simulink library "uav_utilities"  (Simulink 7.1)
values from neighbouring files (symbols this model uses):
  I = find(Ev == Ev(1))    [res_power_junction_m.m]
undefined symbols (not defined in the file or in its folder): euler_0, g, inner_sysd, K_inner, K_outer, Kx_inner, KX_outer, Ky_inner, KY_outer, L, m, omega_0, outer_sysd, pow_gps_pos_sim, pow_gps_vel_sim, pow_imu_pos_sim, pow_imu_rate_sim, pow_sodar_sim, t_comp_inner, t_comp_outer, t_gps, t_imu, t_inner, t_outer, t_sodar, tau, thrust_max, torque_max, Vb_0, XYZ_0
libraries: simulink x33, aero_sim_lib x9, aerolibprivatev1p5 x1
(part 1 of 3)
settings Model: Creator=Administrator  LastModifiedBy=Administrator

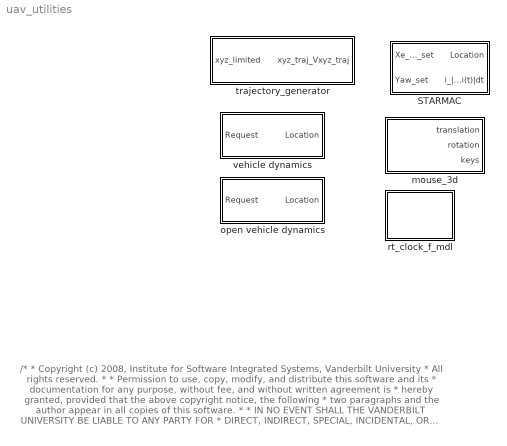
== system uav_utilities ==
  note: /*
      |  * Copyright (c) 2008, Institute for Software Integrated Systems, Vanderbilt University
      |  * All rights reserved.
      |  *
      |  * Permission to use, copy, modify, and distribute this software and its
      |  * documentation for any purpose, without fee, and without written agreement is
      |  * hereby granted, provided that the above copyright notice, the following
      |  * two paragraphs and the author appear in all copies of this software.
      |  *
      |  * IN NO EVENT SHALL THE VANDERBILT UNIVERSITY BE LIABLE TO ANY PARTY FOR
      |  * DIRECT, INDIRECT, SPECIAL, INCIDENTAL, OR CONSEQUENTIAL DAMAGES ARISING OUT
      |  * OF THE USE OF THIS SOFTWARE AND ITS DOCUMENTATION, EVEN IF THE VANDERBILT
      |  * UNIVERSITY HAS BEEN ADVISED OF THE POSSIBILITY OF SUCH DAMAGE.
      |  *
      |  * THE VANDERBILT UNIVERSITY SPECIFICALLY DISCLAIMS ANY WARRANTIES,
      |  * INCLUDING, BUT NOT LIMITED TO, THE IMPLIED WARRANTIES OF MERCHANTABILITY
      |  * AND FITNESS FOR A PARTICULAR PURPOSE.  THE SOFTWARE PROVIDED HEREUNDER IS
      |  * ON AN "AS IS" BASIS, AND THE VANDERBILT UNIVERSITY HAS NO OBLIGATION TO
      |  * PROVIDE MAINTENANCE, SUPPORT, UPDATES, ENHANCEMENTS, OR MODIFICATIONS.
      |  *
      |  * @author Nicholas Kottenstette
      |  */
  STARMAC : Subsystem
  mouse_3d : Subsystem
  open vehicle dynamics : Subsystem  AncestorBlock=uav_utilities/vehicle dynamics
  rt_clock_f_mdl : Subsystem  mask{clock_id=1, T=.01}
      mask prompts: clock_id "Enter clock id (1,2,...) [clock_id]"; T "Enter step time (s) [T]"
      mask init:
      | if clock_id < 1
      |     clock_id = 1;
      | end
      | if T < 0.001
      |     T = .001;
      | end
  trajectory_generator : Subsystem  mask{omega_traj=2*pi/(40*.1), zeta_traj=.9, tau_v_est=.1, T=.01}
      mask prompts: omega_traj "Enter omega trajectory"; zeta_traj "Enter zeta trajectory"; tau_v_est "Enter tau_v_est"; T "Sample time (-1 for inherited):"
      mask init:
      | Hs_x=tf([omega_traj^2],[1 2*zeta_traj*omega_traj omega_traj^2]);
      | Hs_v=tf([1 0],[tau_v_est 1]);
      | Hz_x=ipesh_transform(Hs_x,T);
      | Hz_v=ipesh_transform(Hs_v,T);
  vehicle dynamics : Subsystem

== system uav_utilities/STARMAC ==
  Xe_Ve_set : Inport  PortDimensions=[6]
  Yaw_set : Inport  Port=2  PortDimensions=[1]
  3DM_GX1 : Subsystem  Orientation=left  mask{a_g_s=7000, g_max=5, g_g_s=8500, omega_max=300, Ts=.01}
      mask prompts: a_g_s "AccelGainScale:"; g_max "Max G (1 G = 9.81 m/s^2):"; g_g_s "GyroGainScale:"; omega_max "Mav Angular Velocity (deg/sec):"; Ts "Sample Rate (seconds):"
  Data Type Conversion : DataTypeConversion  OutDataType=sfix(16)  OutScaling=2^0
  Data Type Conversion1 : DataTypeConversion  OutDataType=sfix(16)  OutScaling=2^0
  Demux : Demux  Outputs=[3,3]
  Mux : Mux  Inputs=[3 3 3]
  Rate Transition2 : RateTransition
  SUPERSTAR_II : Subsystem  Orientation=left  mask{Ts=.01}
      mask prompts: Ts "Sample Rate (seconds):"
  Terminator : Terminator
  ZOH : ZeroOrderHold  SampleTime=.01
  ZOH4 : ZeroOrderHold  SampleTime=.01
  Zero-Order Hold : ZeroOrderHold  SampleTime=.02
  dtc : DataTypeConversion  OutDataTypeMode=double  OutDataType=sfix(16)  OutScaling=2^0  OutDataTypeStr=double
  gravity_effects : Constant  Value=zeros(3,1)  OutDataTypeMode=double  OutDataType=sfix(16)  OutScaling=2^0  OutDataTypeStr=double
  gum_stix : Subsystem
  robo_stix : Subsystem  Orientation=left
  starmac_dynamics : Subsystem  AncestorBlock=aero_sim_lib/starmac_dynamics
  Location : Outport
  i_|P_i(t)|dt : Outport  Port=2
  wires:
  ZOH/1 -> Data Type Conversion/1
  robo_stix/5(Ve) -> gum_stix/4(Ve)
  robo_stix/4(Xe) -> gum_stix/3(Xe)
  robo_stix/3(Ab) -> gum_stix/2(Ab)
  Rate Transition2/1 -> dtc/1
  Zero-Order Hold/1 -> Rate Transition2/1
  starmac_dynamics/5(omega) -> 3DM_GX1/3(omega_c)
  dtc/1 -> starmac_dynamics/1(desired_motor_thrust)
  Data Type Conversion/1 -> gum_stix/5(Xe_set)
  gum_stix/2(u_euler) -> robo_stix/4(euler_set)
  gum_stix/1(u_T) -> robo_stix/5(u_T)
  gravity_effects/1 -> starmac_dynamics/2(wind_velocity)
  starmac_dynamics/1(Ve) -> Mux/2, SUPERSTAR_II/2(Ve)  "Ve"
  starmac_dynamics/2(Xe) -> Mux/1, SUPERSTAR_II/1(Xe)  "Xe"
  SUPERSTAR_II/2(Ve_s) -> robo_stix/7(Ve_s)
  SUPERSTAR_II/1(Xe_s) -> robo_stix/6(Xe_s)
  robo_stix/2(euler1) -> gum_stix/1(euler)
  3DM_GX1/3(omega_s) -> robo_stix/3(omega_s)
  3DM_GX1/2(Ab_s) -> robo_stix/2(Ab_s)
  3DM_GX1/1(euler_s) -> robo_stix/1(euler_s)
  starmac_dynamics/7(Ab) -> 3DM_GX1/2(Ab_c)
  starmac_dynamics/3(euler) -> Mux/3, 3DM_GX1/1(euler_c)  "euler"
  robo_stix/1(cont_motor_thrust) -> Zero-Order Hold/1
  Mux/1 -> Location/1
  Xe_Ve_set/1 -> Demux/1
  Demux/1 -> ZOH/1
  Demux/2 -> Terminator/1
  Yaw_set/1 -> ZOH4/1
  ZOH4/1 -> Data Type Conversion1/1
  Data Type Conversion1/1 -> gum_stix/6(Yaw_set)
  starmac_dynamics/8(i_|P_i(t)|dt) -> i_|P_i(t)|dt/1

== system uav_utilities/mouse_3d ==
  Demux : Demux  Outputs=[3,3,-1]
  Gain4 : Gain  Gain=.003  ParameterDataType=sfix(16)  ParameterScaling=2^0  OutDataType=sfix(16)  OutScaling=2^0
  mouse_3d : S-Function  FunctionName=mouse_3d  EnableBusSupport=off
  translation : Outport  OutDataType=sfix(16)  OutScaling=2^0
  rotation : Outport  Port=2  OutDataType=sfix(16)  OutScaling=2^0
  keys : Outport  Port=3  OutDataType=sfix(16)  OutScaling=2^0
  wires:
  Demux/2 -> rotation/1
  Demux/1 -> Gain4/1
  mouse_3d/1 -> Demux/1
  Gain4/1 -> translation/1
  Demux/3 -> keys/1

== system uav_utilities/open vehicle dynamics ==
  note: STARMAC Vehicle Model
  Request : Inport  OutDataType=sfix(16)  OutScaling=2^0
  Angular Rates : ToWorkspace  VariableName=pqr1  SampleTime=-1  SaveFormat=Array
  Body Velocity : ToWorkspace  VariableName=Vb1  SampleTime=-1  SaveFormat=Array
  Clock : Clock
      settings: Decimation=10
  Demux : Demux  Outputs=3
  Demux1 : Demux  Outputs=3
  Demux2 : Demux  Outputs=3
  Demux3 : Demux  Outputs=6
  Euler Angles : ToWorkspace  VariableName=eulerout1  SampleTime=-1  SaveFormat=Array
  Inner Loop : Subsystem
  Mux : Mux  Inputs=9
  Mux1 : Mux  Inputs=3
  Mux2 : Mux  Inputs=3
  Outer Loop Controller : Subsystem
  Position : ToWorkspace  VariableName=xout1  SampleTime=-1  SaveFormat=Array
  Scope : Scope  NumInputPorts=3
      settings: TimeRange=9  YMin=-1~-0.9~-0.65  YMax=1~0.3~0.05  SaveName=ScopeData15  Decimation=10
  Time : ToWorkspace  VariableName=time1  SampleTime=-1  SaveFormat=Array
  Velocity : ToWorkspace  VariableName=vout1  SampleTime=-1  SaveFormat=Array
  Location : Outport  OutDataType=sfix(16)  OutScaling=2^0
  wires:
  Outer Loop Controller/1(Outer Loop Request) -> Inner Loop/1(Outer Loop Request)
  Inner Loop/3(Velocity) -> Outer Loop Controller/3(Velocity), Velocity/1, Demux1/1
  Inner Loop/1(Body vel) -> Body Velocity/1
  Inner Loop/4(Angular Rates) -> Angular Rates/1
  Inner Loop/5(Euler Angles) -> Euler Angles/1, Demux2/1
  Clock/1 -> Time/1
  Inner Loop/6(Inner Loop State) -> Outer Loop Controller/4(Inner Loop  State)
  Demux/1 -> Mux/1
  Demux/2 -> Mux/2
  Demux/3 -> Mux/3
  Demux1/1 -> Mux/4
  Demux1/2 -> Mux/5
  Demux1/3 -> Mux/6
  Demux2/1 -> Mux/7
  Demux2/2 -> Mux/8
  Demux2/3 -> Mux/9
  Demux3/4 -> Mux2/1  "xdot_c"
  Demux3/5 -> Mux2/2  "ydot_c"
  Demux3/6 -> Mux2/3  "zdot_c"
  Demux3/3 -> Mux1/3  "z_c"
  Demux3/1 -> Mux1/1  "x_c"
  Demux3/2 -> Mux1/2  "y_c"
  Mux2/1 -> Scope/1  "speed req"
  Mux1/1 -> Scope/2  "requested location"
  Mux/1 -> Location/1
  Request/1 -> Outer Loop Controller/1(Request), Demux3/1
  Inner Loop/2(Position) -> Position/1, Demux/1, Scope/3, Outer Loop Controller/2(Position)  "curr pos"

== system uav_utilities/rt_clock_f_mdl ==
  force_rate : Scope
      settings: YMin=-7.5  YMax=7.5  SaveName=ScopeData4  MaxDataPoints=100
  rt_clock_f_mdl_in : S-Function  FunctionName=rt_clock_f  Parameters=clock_id,T  EnableBusSupport=off
  wires:
  rt_clock_f_mdl_in/1 -> force_rate/1

== system uav_utilities/trajectory_generator ==
  xyz_limited : Inport  OutDataType=sfix(16)  OutScaling=2^0
  Demux9 : Demux  Outputs=3
  Mux1 : Mux  Inputs=3
  Mux2 : Mux  Inputs=3
  Mux3 : Mux  Inputs=2
  Zero-Order Hold : ZeroOrderHold  SampleTime=T
  Zero-Order Hold1 : ZeroOrderHold  SampleTime=T
  Zero-Order Hold2 : ZeroOrderHold  SampleTime=T
  v_xyz_traj : DiscreteTransferFcn  Numerator=Hz_v.num{1}  Denominator=Hz_v.den{1}  SampleTime=T
  v_xyz_traj1 : DiscreteTransferFcn  Numerator=Hz_v.num{1}  Denominator=Hz_v.den{1}  SampleTime=T
  v_xyz_traj2 : DiscreteTransferFcn  Numerator=Hz_v.num{1}  Denominator=Hz_v.den{1}  SampleTime=T
  xyz_traj : DiscreteTransferFcn  Numerator=Hz_x.num{1}  Denominator=Hz_x.den{1}  SampleTime=T
  xyz_traj1 : DiscreteTransferFcn  Numerator=Hz_x.num{1}  Denominator=Hz_x.den{1}  SampleTime=T
  xyz_traj2 : DiscreteTransferFcn  Numerator=Hz_x.num{1}  Denominator=Hz_x.den{1}  SampleTime=T
  xyz_traj_Vxyz_traj : Outport  OutDataType=sfix(16)  OutScaling=2^0
  wires:
  Mux3/1 -> xyz_traj_Vxyz_traj/1
  Zero-Order Hold2/1 -> Mux3/2
  Zero-Order Hold1/1 -> Mux3/1
  Zero-Order Hold/1 -> Demux9/1
  Mux2/1 -> Zero-Order Hold2/1
  Mux1/1 -> Zero-Order Hold1/1
  xyz_limited/1 -> Zero-Order Hold/1
  v_xyz_traj2/1 -> Mux2/3
  v_xyz_traj/1 -> Mux2/1
  v_xyz_traj1/1 -> Mux2/2
  xyz_traj2/1 -> Mux1/3, v_xyz_traj2/1
  xyz_traj1/1 -> Mux1/2, v_xyz_traj1/1
  xyz_traj/1 -> Mux1/1, v_xyz_traj/1
  Demux9/3 -> xyz_traj2/1
  Demux9/2 -> xyz_traj1/1
  Demux9/1 -> xyz_traj/1

== system uav_utilities/vehicle dynamics ==
  note: STARMAC Vehicle Model
  Request : Inport
  Angular Rates : ToWorkspace  VariableName=pqr1  SampleTime=-1  SaveFormat=Array
  Body Velocity : ToWorkspace  VariableName=Vb1  SampleTime=-1  SaveFormat=Array
  Clock : Clock
      settings: Decimation=10
  Demux : Demux  Outputs=3
  Demux1 : Demux  Outputs=3
  Demux2 : Demux  Outputs=3
  Demux3 : Demux  Outputs=6
  Euler Angles : ToWorkspace  VariableName=eulerout1  SampleTime=-1  SaveFormat=Array
  Inner Loop : Subsystem
  Mux : Mux  Inputs=9
  Mux1 : Mux  Inputs=3
  Mux2 : Mux  Inputs=3
  Outer Loop Controller : Subsystem
  Position : ToWorkspace  VariableName=xout1  SampleTime=-1  SaveFormat=Array
  Scope : Scope  NumInputPorts=3
      settings: TimeRange=9  YMin=-1~-0.9~-0.65  YMax=1~0.3~0.05  SaveName=ScopeData15  Decimation=10
  Time : ToWorkspace  VariableName=time1  SampleTime=-1  SaveFormat=Array
  Velocity : ToWorkspace  VariableName=vout1  SampleTime=-1  SaveFormat=Array
  Location : Outport
  wires:
  Inner Loop/2(Position) -> Outer Loop Controller/2(Position), Scope/3, Demux/1, Position/1  "curr pos"
  Request/1 -> Demux3/1, Outer Loop Controller/1(Request)
  Mux/1 -> Location/1
  Mux1/1 -> Scope/2  "requested location"
  Mux2/1 -> Scope/1  "speed req"
  Demux3/2 -> Mux1/2  "y_c"
  Demux3/1 -> Mux1/1  "x_c"
  Demux3/3 -> Mux1/3  "z_c"
  Demux3/6 -> Mux2/3  "zdot_c"
  Demux3/5 -> Mux2/2  "ydot_c"
  Demux3/4 -> Mux2/1  "xdot_c"
  Demux2/3 -> Mux/9
  Demux2/2 -> Mux/8
  Demux2/1 -> Mux/7
  Demux1/3 -> Mux/6
  Demux1/2 -> Mux/5
  Demux1/1 -> Mux/4
  Demux/3 -> Mux/3
  Demux/2 -> Mux/2
  Demux/1 -> Mux/1
  Inner Loop/6(Inner Loop State) -> Outer Loop Controller/4(Inner Loop  State)
  Clock/1 -> Time/1
  Inner Loop/5(Euler Angles) -> Demux2/1, Euler Angles/1
  Inner Loop/4(Angular Rates) -> Angular Rates/1
  Inner Loop/1(Body vel) -> Body Velocity/1
  Inner Loop/3(Velocity) -> Demux1/1, Velocity/1, Outer Loop Controller/3(Velocity)
  Outer Loop Controller/1(Outer Loop Request) -> Inner Loop/1(Outer Loop Request)

== system uav_utilities/STARMAC/3DM_GX1 ==
  euler_c : Inport  Orientation=left
  Ab_c : Inport  Orientation=left  Port=2
  omega_c : Inport  Orientation=left  Port=3
  Demux : Demux  Orientation=left  Outputs=[3 3 3]
  Mux : Mux  Orientation=left  Inputs=[3 3 3]
  Quantizer : Quantizer  Orientation=left  QuantizationInterval=pi/(2^15)*ones(3,1)
  Quantizer1 : Quantizer  Orientation=left  QuantizationInterval=g_max*9.81/(2^15)*ones(3,1)
  Quantizer2 : Quantizer  Orientation=left  QuantizationInterval=(pi*omega_max/180)/(2^15)*ones(3,1)
  Saturation : Saturate  Orientation=left  UpperLimit=((2^15)-1)*ones(3,1)  LowerLimit=-(2^15)*ones(3,1)  OutDataType=sfix(16)  OutScaling=2^0
  Saturation1 : Saturate  Orientation=left  UpperLimit=((2^15)-1)*ones(3,1)  LowerLimit=-(2^15)*ones(3,1)  OutDataType=sfix(16)  OutScaling=2^0
  Zero-Order Hold : ZeroOrderHold  Orientation=left  SampleTime=Ts
  counts_per_accel : Gain  Orientation=left  Gain=1e3*(2^15)/(9.81*a_g_s)  ParameterDataType=sfix(16)  ParameterScaling=2^0  OutDataType=sfix(16)  OutScaling=2^0
  counts_per_radian : Gain  Orientation=left  Gain=(2^15)/pi  ParameterDataType=sfix(16)  ParameterScaling=2^0  OutDataType=sfix(16)  OutScaling=2^0
  counts_per_radian_p_sec : Gain  Orientation=left  Gain=1e3*(2^15)/g_g_s  ParameterDataType=sfix(16)  ParameterScaling=2^0  OutDataType=sfix(16)  OutScaling=2^0
  dtc1 : DataTypeConversion  Orientation=left  OutDataTypeMode=single  OutDataType=sfix(16)  OutScaling=2^0  OutDataTypeStr=single
  dtc2 : DataTypeConversion  Orientation=left  OutDataTypeMode=single  OutDataType=sfix(16)  OutScaling=2^0  OutDataTypeStr=single
  dtc3 : DataTypeConversion  Orientation=left  OutDataTypeMode=single  OutDataType=sfix(16)  OutScaling=2^0  OutDataTypeStr=single
  euler_s : Outport  Orientation=left
  Ab_s : Outport  Orientation=left  Port=2
  omega_s : Outport  Orientation=left  Port=3
  wires:
  counts_per_radian/1 -> dtc1/1
  dtc3/1 -> omega_s/1
  dtc2/1 -> Ab_s/1
  dtc1/1 -> euler_s/1
  Saturation1/1 -> dtc3/1
  Saturation/1 -> dtc2/1
  Quantizer2/1 -> counts_per_radian_p_sec/1
  counts_per_radian_p_sec/1 -> Saturation1/1
  Demux/3 -> Quantizer2/1
  counts_per_accel/1 -> Saturation/1
  Quantizer1/1 -> counts_per_accel/1
  Quantizer/1 -> counts_per_radian/1
  Demux/2 -> Quantizer1/1
  Demux/1 -> Quantizer/1
  Zero-Order Hold/1 -> Demux/1
  omega_c/1 -> Mux/3
  Ab_c/1 -> Mux/2
  euler_c/1 -> Mux/1
  Mux/1 -> Zero-Order Hold/1

== system uav_utilities/STARMAC/SUPERSTAR_II ==
  Xe : Inport  Orientation=left
  Ve : Inport  Orientation=left  Port=2
  Demux : Demux  Orientation=left  Outputs=[3 3]
  Mux : Mux  Orientation=left  Inputs=[3 3]
  Rate Transition : RateTransition  Orientation=left
  ZOH : ZeroOrderHold  Orientation=left  SampleTime=Ts
  dtc1 : DataTypeConversion  Orientation=left  OutDataTypeMode=single  OutDataType=sfix(16)  OutScaling=2^0  OutDataTypeStr=single
  dtc2 : DataTypeConversion  Orientation=left  OutDataTypeMode=single  OutDataType=sfix(16)  OutScaling=2^0  OutDataTypeStr=single
  Xe_s : Outport  Orientation=left
  Ve_s : Outport  Orientation=left  Port=2
  wires:
  Rate Transition/1 -> Demux/1
  dtc2/1 -> Ve_s/1
  dtc1/1 -> Xe_s/1
  Demux/2 -> dtc2/1
  Demux/1 -> dtc1/1
  Mux/1 -> ZOH/1
  Xe/1 -> Mux/1
  Ve/1 -> Mux/2
  ZOH/1 -> Rate Transition/1

== system uav_utilities/STARMAC/gum_stix ==
  euler : Inport  PortDimensions=[3]  DataType=single  OutDataTypeStr=single
  Ab : Inport  Port=2  PortDimensions=[3]  DataType=single  OutDataTypeStr=single
  Xe : Inport  Port=3  PortDimensions=[3]  DataType=single  OutDataTypeStr=single
  Ve : Inport  Port=4  PortDimensions=[3]  DataType=single  OutDataTypeStr=single
  Xe_set : Inport  Port=5  PortDimensions=[3]  DataType=single  OutDataTypeStr=single
  Yaw_set : Inport  Port=6  PortDimensions=[1]  DataType=single  OutDataTypeStr=single
  Demux : Demux  Outputs=3
  body_to_inertial : Subsystem
  inertial_pos_controller : Subsystem
  rate_limiter : Subsystem  mask{wn=2*pi, zeta=0.9, Vmax=2, T=0.01}
      mask prompts: wn "omega_n"; Vmax "Max velocity"; T "Sample time"
      mask init:
      | Hs=tf([wn^2],[1,2*zeta*wn,wn^2]);
      | Hz=ipesh_transform(Hs,T);
  sc1 : Scope
      settings: YMin=-7.5  YMax=22.5  SaveName=ScopeData8  Decimation=10
  sc2 : Scope
      settings: YMin=-2  YMax=2  SaveName=ScopeData9  Decimation=10
  sensor_fusion : Subsystem
  u_T : Outport  PortDimensions=[1]  DataType=single  OutDataTypeStr=single
  u_euler : Outport  Port=2  PortDimensions=[3]  DataType=single  OutDataTypeStr=single
  wires:
  Yaw_set/1 -> inertial_pos_controller/5(Yaw_set)
  Demux/3 -> inertial_pos_controller/4(Yaw_actual)
  rate_limiter/1(Xr_set) -> sc2/1, inertial_pos_controller/1(Xe_set)
  Ve/1 -> sensor_fusion/4(Ve_s)
  Xe/1 -> sensor_fusion/3(Xe_s)
  body_to_inertial/2(Ve) -> sensor_fusion/2(Ve_f)
  body_to_inertial/1(Xe) -> sensor_fusion/1(Xe_f)
  sensor_fusion/2(Ve) -> inertial_pos_controller/3(Ve)
  sensor_fusion/1(Xe) -> inertial_pos_controller/2(Xe)
  Ab/1 -> body_to_inertial/2(Ab)
  euler/1 -> Demux/1, body_to_inertial/1(euler)
  inertial_pos_controller/2(u_euler) -> u_euler/1
  inertial_pos_controller/1(u_T) -> u_T/1
  Xe_set/1 -> sc1/1, rate_limiter/1(Xe_set)

== system uav_utilities/STARMAC/robo_stix ==
  euler_s : Inport  PortDimensions=[3]  DataType=single  OutDataTypeStr=single
  Ab_s : Inport  Port=2  PortDimensions=[3]  DataType=single  OutDataTypeStr=single
  omega_s : Inport  Port=3  PortDimensions=[3]  DataType=single  OutDataTypeStr=single
  euler_set : Inport  Port=4  PortDimensions=[3]  DataType=single  OutDataTypeStr=single
  u_T : Inport  Port=5  PortDimensions=[1]  DataType=single  OutDataTypeStr=single
  Xe_s : Inport  Port=6  PortDimensions=[3]  DataType=single  OutDataTypeStr=single
  Ve_s : Inport  Port=7  PortDimensions=[3]  DataType=single  OutDataTypeStr=single
  euler_controller : Subsystem  mask{K=1, K_e=7.5/.65, K_o=.5}
      mask prompts: K "Loop Gain [K]:"; K_e "Euler Gain [K_e]:"; K_o "Omega Gain [K_o]:"
  lead_motor : Subsystem  mask{tau_motor=.10, t_s=.01}
      mask init:
      | Hs=tf([tau_motor 1],[t_s/pi 1]);
      | Hz=ipesh_transform(Hs,t_s);
      | %a=1/tau_motor;
      | %b=pi/t_s;
      | %T=t_s;
      | %num1=b*(1-exp(-b*T))+a*(b*T-1+exp(-b*T));
      | %num2=-b*(1-exp(-b*T))+a*(1-exp(-b*T)-b*T*exp(-b*T));
      | %den1=a*b;
      | %den2=-a*b*exp(-b*T);
      | %num=[num1 num2];
      | %den=[den1 den2];
      | %Hz=tf(num,den,T);
      | %[y,t]=step(Hz);
      | %k_ss=(1/y(length(y)));
      | %num=k_ss*num;
      | %lead_a_1=single(-den(2)/den(1))
      | %lead_b_1=single(num(2)/den(1))
      | %lead_b_2=single(num(1)/den(1))
      | %Hz=k_ss*Hz
      | %bode(Hz);
  sensor_convert : Subsystem  mask{a_g_s=7000, g_g_s=8500}
      mask prompts: a_g_s "AccelGainScale[a_g_s]:"; g_g_s "GyroGainScale[g_g_s]:"
  thrust_limit : Saturate  UpperLimit=10*ones(4,1)  LowerLimit=0*ones(4,1)  OutDataTypeMode=single  OutDataType=sfix(16)  OutScaling=2^0  OutDataTypeStr=single
  u_T_u_torque_motor_thrust : Subsystem  mask{dx=.3048, K_torque=.47}
      mask prompts: dx "X distance of motor from CG [dx](meters):"; K_torque "Ktorque [K_torque]:"
      mask init:
      | M=[0 -dx 0 dx;
      |    dx 0 -dx 0;
      |    -K_torque K_torque -K_torque K_torque;
      |    1 1 1 1];
      | Mi=single(inv(M));
  cont_motor_thrust : Outport
  euler1 : Outport  Port=2
  Ab : Outport  Port=3
  Xe : Outport  Port=4
  Ve : Outport  Port=5
  wires:
  lead_motor/1(thrust_out) -> thrust_limit/1
  u_T_u_torque_motor_thrust/1(cont_motor_thrust) -> lead_motor/1(thrust_in)
  Xe_s/1 -> Xe/1
  thrust_limit/1 -> cont_motor_thrust/1
  Ve_s/1 -> Ve/1
  sensor_convert/2(Ab) -> Ab/1
  euler_controller/1(u_torque) -> u_T_u_torque_motor_thrust/1(u_torque)
  u_T/1 -> u_T_u_torque_motor_thrust/2(u_T)
  sensor_convert/3(omega) -> euler_controller/3(omega)
  euler_set/1 -> euler_controller/1(euler_set)
  sensor_convert/1(euler) -> euler1/1, euler_controller/2(euler)
  omega_s/1 -> sensor_convert/3(omega_s)
  Ab_s/1 -> sensor_convert/2(Ab_s)
  euler_s/1 -> sensor_convert/1(euler_s)

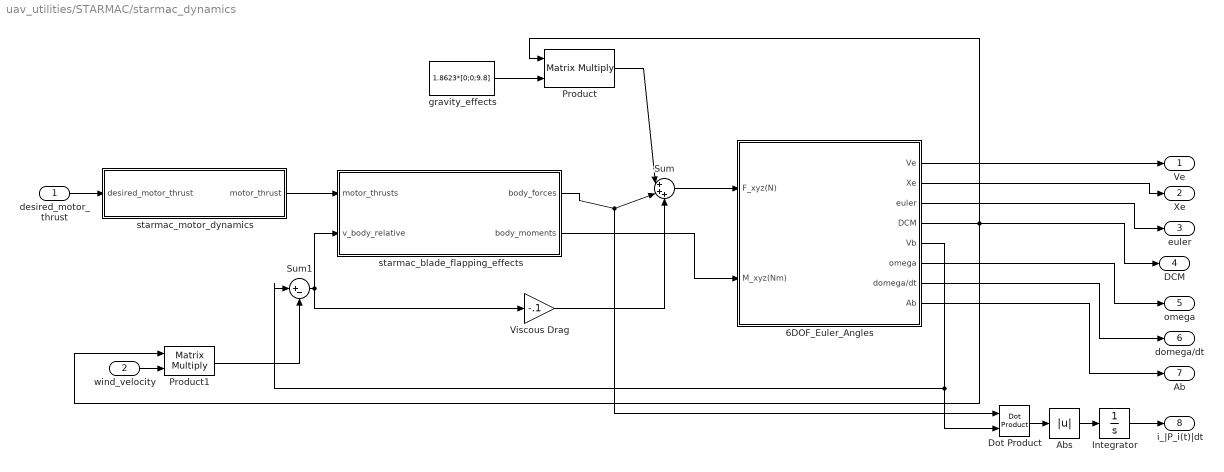
== system uav_utilities/STARMAC/starmac_dynamics ==
  desired_motor_thrust : Inport  OutDataType=sfix(16)  OutScaling=2^0
  wind_velocity : Inport  Port=2  OutDataType=sfix(16)  OutScaling=2^0
  6DOF_Euler_Angles : Subsystem  AncestorBlock=aero_sim_lib/6DOF (Euler Angles)_CMU  mask{XYZe_0=[0.1;0.2;0], Vb_0=[0;0;0], euler_0=[0;0;0], omega_0=[0;0;0], M=1.8623, I=diag([0.02759 0.02771 0.04806])}
      mask prompts: XYZe_0 "Initial position in inertial axes [Xe,Ye,Ze]:"; Vb_0 "Initial velocity in body axes [U,v,w]:"; euler_0 "Initial Euler orientation [roll, pitch, yaw]=[phi,theta,psi]:"; omega_0 "Initial body rotation rates [p,q,r]=omega:"; M "Initial mass:"; I "Inertial:"
  Abs : Abs  OutDataType=sfix(16)  OutScaling=2^0
  Dot Product : simulink/Math Operations/Dot Product  InputSameDT=on  OutDataType=sfix(16)  OutScaling=2^-10  DoSatur=off
  Integrator : Integrator
  Product : Product  Multiplication=Matrix(*)  OutDataType=sfix(16)  OutScaling=2^0  RndMeth=Zero
  Product1 : Product  Multiplication=Matrix(*)  OutDataType=sfix(16)  OutScaling=2^0  RndMeth=Zero
  Sum : Sum  Inputs=|+++  OutDataType=sfix(16)  OutScaling=2^0
  Sum1 : Sum  Inputs=|+-  OutDataType=sfix(16)  OutScaling=2^0
  Viscous Drag : Gain  Gain=-.1  ParameterDataType=sfix(16)  ParameterScaling=2^0  OutDataType=sfix(16)  OutScaling=2^0
  gravity_effects : Constant  Value=1.8623*[0;0;9.8]  OutDataType=sfix(16)  OutScaling=2^0
  starmac_blade_flapping_effects : Subsystem  AncestorBlock=aero_sim_lib/starmac_blade_flapping_effects
  starmac_motor_dynamics : Subsystem  AncestorBlock=aero_sim_lib/starmac_motor_dynamics  mask{tau_motor=.1, T_nom=1.8263*9.8/4, thrust_max=9.8, thrust_min=0, motor_lag_enable=on, motor_variance=.01*(.05*9.8/4)^2, Ts=1/76}
      mask prompts: tau_motor "tau_motor (seconds):"; T_nom "nominal thrust (N):"; thrust_max "maximum thrust (N):"; thrust_min "minimum thrust (N):"; motor_lag_enable "Motor Lag Enabled:"; motor_variance "Motor Variance [motor_variance]:"; Ts "Motor Update Rate (seconds):"
  Ve : Outport  OutDataType=sfix(16)  OutScaling=2^0
  Xe : Outport  Port=2  OutDataType=sfix(16)  OutScaling=2^0
  euler : Outport  Port=3  OutDataType=sfix(16)  OutScaling=2^0
  DCM : Outport  Port=4  OutDataType=sfix(16)  OutScaling=2^0
  omega : Outport  Port=5  OutDataType=sfix(16)  OutScaling=2^0
  domega/dt : Outport  Port=6  OutDataType=sfix(16)  OutScaling=2^0
  Ab : Outport  Port=7  OutDataType=sfix(16)  OutScaling=2^0
  i_|P_i(t)|dt : Outport  Port=8  OutDataType=sfix(16)  OutScaling=2^0
  wires:
  Abs/1 -> Integrator/1
  Dot Product/1 -> Abs/1
  Integrator/1 -> i_|P_i(t)|dt/1
  6DOF_Euler_Angles/8(Ab) -> Ab/1
  6DOF_Euler_Angles/7(domega/dt) -> domega/dt/1
  6DOF_Euler_Angles/6(omega) -> omega/1
  6DOF_Euler_Angles/3(euler) -> euler/1
  6DOF_Euler_Angles/2(Xe) -> Xe/1
  6DOF_Euler_Angles/1(Ve) -> Ve/1
  starmac_motor_dynamics/1(motor_thrust) -> starmac_blade_flapping_effects/1(motor_thrusts)
  Product/1 -> Sum/1
  Sum/1 -> 6DOF_Euler_Angles/1(F_xyz(N))
  6DOF_Euler_Angles/4(DCM) -> DCM/1, Product/1, Product1/1
  gravity_effects/1 -> Product/2
  Sum1/1 -> starmac_blade_flapping_effects/2(v_body_relative), Viscous Drag/1
  Product1/1 -> Sum1/2
  6DOF_Euler_Angles/5(Vb) -> Dot Product/2, Sum1/1
  Viscous Drag/1 -> Sum/3
  starmac_blade_flapping_effects/2(body_moments) -> 6DOF_Euler_Angles/2(M_xyz(Nm))
  starmac_blade_flapping_effects/1(body_forces) -> Dot Product/1, Sum/2
  desired_motor_thrust/1 -> starmac_motor_dynamics/1(desired_motor_thrust)
  wind_velocity/1 -> Product1/2

== system uav_utilities/open vehicle dynamics/Inner Loop ==
  note: Inner Loop Model
  note: \phi,\theta,\psi,p,q,r
  note: \phi,\theta,\psi
  Outer Loop Request : Inport  OutDataType=sfix(16)  OutScaling=2^0
  Attitude Request : ToWorkspace  VariableName=eulreq1  SampleTime=-1  SaveFormat=Array
  Demux1 : Demux  Orientation=left  Outputs=3
  Inner Loop Controller : Subsystem
  Mux1 : Mux  Orientation=left  Inputs=2
  Non-Linear Dynamics : Subsystem
  Saturation : Subsystem
  attitude : Scope
      settings: YMin=-4  YMax=10  SaveName=ScopeData4
  pqr : Scope
      settings: YMin=-4  YMax=10  SaveName=ScopeData3
  velocity : Scope
      settings: YMin=-4  YMax=10  SaveName=ScopeData2
  x : Terminator
  xyz : Scope
      settings: YMin=-0.1  YMax=1.2
  y : Terminator
  Body vel : Outport  OutDataType=sfix(16)  OutScaling=2^0
  Position : Outport  Port=2  OutDataType=sfix(16)  OutScaling=2^0
  Velocity : Outport  Port=3  OutDataType=sfix(16)  OutScaling=2^0
  Angular Rates : Outport  Port=4  OutDataType=sfix(16)  OutScaling=2^0
  Euler Angles : Outport  Port=5  OutDataType=sfix(16)  OutScaling=2^0
  Inner Loop State : Outport  Port=6  OutDataType=sfix(16)  OutScaling=2^0
  wires:
  Non-Linear Dynamics/2(Position) -> Demux1/1, xyz/1, Saturation/1(Actual)  "x,y,z"
  Non-Linear Dynamics/1("Body vel ") -> Body vel/1
  Inner Loop Controller/1(Thrust Command) -> Non-Linear Dynamics/1(Thrust Command 1-4)
  Non-Linear Dynamics/5(Euler Angles) -> Euler Angles/1, Mux1/1, attitude/1
  Non-Linear Dynamics/4(Angular Rates) -> Angular Rates/1, Mux1/2, pqr/1  "p,q,r"
  Non-Linear Dynamics/3(Velocity) -> Velocity/1, velocity/1  "xdot,ydot,zdot"
  Mux1/1 -> Inner Loop Controller/2(Attitude State)
  Demux1/3 -> Inner Loop Controller/3(z State)
  Demux1/2 -> x/1
  Demux1/1 -> y/1
  Outer Loop Request/1 -> Inner Loop Controller/1(Outer Loop Request), Attitude Request/1
  Saturation/1(Sensed) -> Position/1
  Inner Loop Controller/2(Inner Loop State) -> Inner Loop State/1

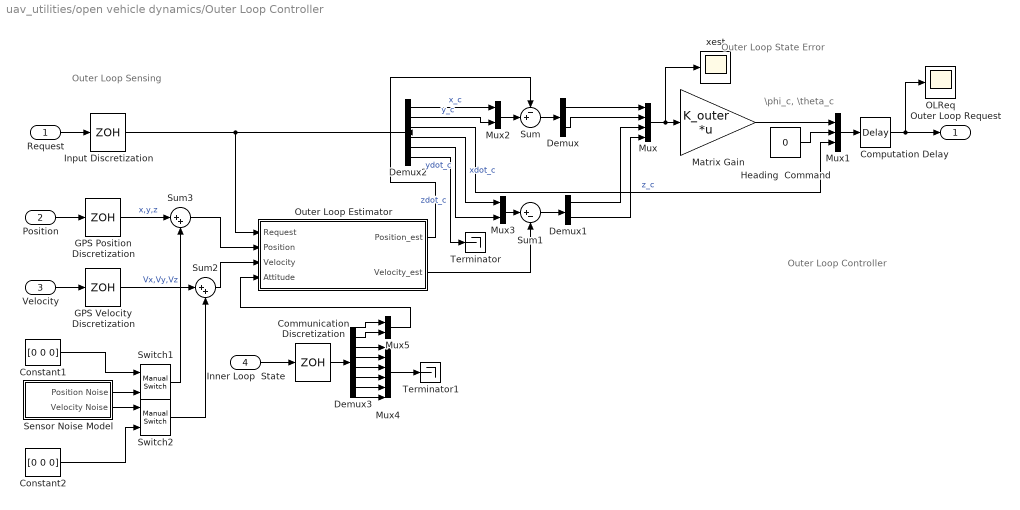
== system uav_utilities/open vehicle dynamics/Outer Loop Controller ==
  note: Outer Loop Controller
  note: \phi_c, \theta_c
  note: Outer Loop
      | State Error
  note: Outer Loop Sensing
  Request : Inport  OutDataType=sfix(16)  OutScaling=2^0
  Position : Inport  Port=2  OutDataType=sfix(16)  OutScaling=2^0
  Velocity : Inport  Port=3  OutDataType=sfix(16)  OutScaling=2^0
  Inner Loop  State : Inport  Port=4  OutDataType=sfix(16)  OutScaling=2^0
  Communication Discretization : ZeroOrderHold  SampleTime=t_outer
  Computation Delay : TransportDelay  DelayTime=t_comp_outer
  Constant1 : Constant  Value=[0 0 0]  OutDataType=sfix(16)  OutScaling=2^0
  Constant2 : Constant  Value=[0 0 0]  OutDataType=sfix(16)  OutScaling=2^0
  Demux : Demux  Outputs=2
  Demux1 : Demux  Outputs=2
  Demux2 : Demux  Outputs=6
  Demux3 : Demux  Outputs=8
  GPS Position Discretization : ZeroOrderHold  SampleTime=t_gps
  GPS Velocity Discretization : ZeroOrderHold  SampleTime=t_gps
  Heading  Command : Constant  Value=0  OutDataType=sfix(16)  OutScaling=2^0
  Input Discretization : ZeroOrderHold  SampleTime=t_outer
  Matrix Gain : Gain  Gain=K_outer  Multiplication=Matrix(K*u)  ParameterDataType=sfix(16)  ParameterScaling=2^0  OutDataType=sfix(16)  OutScaling=2^0  SaturateOnIntegerOverflow=on  OutDataTypeStr=Inherit: Same as input  ParamDataTypeStr=Inherit: Same as input
  Mux : Mux
  Mux1 : Mux  Inputs=3
  Mux2 : Mux  Inputs=2
  Mux3 : Mux  Inputs=2
  Mux4 : Mux  Inputs=6
  Mux5 : Mux  Inputs=2
  OLReq : Scope
      settings: YMin=-0.1  YMax=2  SaveName=ScopeData6
  Outer Loop Estimator : Subsystem
  "Sensor Noise Model " : Subsystem
  Sum : Sum  Inputs=-+|  OutDataType=sfix(16)  OutScaling=2^0  SaturateOnIntegerOverflow=on
  Sum1 : Sum  Inputs=|+-  OutDataType=sfix(16)  OutScaling=2^0  SaturateOnIntegerOverflow=on
  Sum2 : Sum  Inputs=|++  OutDataType=sfix(16)  OutScaling=2^0  SaturateOnIntegerOverflow=on
  Sum3 : Sum  Inputs=|++  OutDataType=sfix(16)  OutScaling=2^0  SaturateOnIntegerOverflow=on
  Switch1 : simulink/Signal Routing/Manual Switch  SystemSampleTime=-1  sw=1  action=0  varsize=off
  Switch2 : simulink/Signal Routing/Manual Switch  SystemSampleTime=-1  sw=0  action=0  varsize=off
  Terminator : Terminator
  Terminator1 : Terminator
  xest : Scope
      settings: YMin=-0.2  YMax=0.125  SaveName=ScopeData11
  Outer Loop Request : Outport  OutDataType=sfix(16)  OutScaling=2^0
  wires:
  Position/1 -> GPS Position Discretization/1
  Velocity/1 -> GPS Velocity Discretization/1
  Sum1/1 -> Demux1/1
  Sum/1 -> Demux/1
  Demux/1 -> Mux/1
  Demux/2 -> Mux/2
  Demux1/1 -> Mux/3
  Demux1/2 -> Mux/4
  Request/1 -> Input Discretization/1
  Mux3/1 -> Sum1/1
  Demux2/3 -> Mux1/3  "z_c"
  Demux2/4 -> Mux3/1  "xdot_c"
  Demux2/5 -> Mux3/2  "ydot_c"
  Input Discretization/1 -> Demux2/1, Outer Loop Estimator/1(Request)
  Demux2/1 -> Mux2/1  "x_c"
  Demux2/2 -> Mux2/2  "y_c"
  Demux2/6 -> Terminator/1  "zdot_c"
  GPS Position Discretization/1 -> Sum3/1  "x,y,z"
  GPS Velocity Discretization/1 -> Sum2/1  "Vx,Vy,Vz"
  Outer Loop Estimator/2(Velocity_est) -> Sum1/2
  Mux2/1 -> Sum/2
  Outer Loop Estimator/1(Position_est) -> Sum/1
  Matrix Gain/1 -> Mux1/1
  Mux1/1 -> Computation Delay/1
  Computation Delay/1 -> Outer Loop Request/1, OLReq/1
  Heading  Command/1 -> Mux1/2
  Mux/1 -> Matrix Gain/1, xest/1
  Inner Loop  State/1 -> Communication Discretization/1
  Demux3/8 -> Mux4/6
  Demux3/7 -> Mux4/5
  Demux3/6 -> Mux4/4
  Demux3/5 -> Mux4/3
  Demux3/4 -> Mux4/2
  Demux3/3 -> Mux4/1
  Mux4/1 -> Terminator1/1
  Demux3/1 -> Mux5/1
  Demux3/2 -> Mux5/2
  Mux5/1 -> Outer Loop Estimator/4(Attitude)
  Sum2/1 -> Outer Loop Estimator/3(Velocity)
  Sum3/1 -> Outer Loop Estimator/2(Position)
  "Sensor Noise Model "/2(Velocity Noise) -> Switch2/1
  Switch2/1 -> Sum2/2
  "Sensor Noise Model "/1(Position Noise) -> Switch1/2
  Switch1/1 -> Sum3/2
  Constant2/1 -> Switch2/2
  Constant1/1 -> Switch1/1
  Communication Discretization/1 -> Demux3/1

== system uav_utilities/vehicle dynamics/Inner Loop ==
  note: \phi,\theta,\psi
  note: \phi,\theta,\psi,p,q,r
  note: Inner Loop Model
  Outer Loop Request : Inport
  Attitude Request : ToWorkspace  VariableName=eulreq1  SampleTime=-1  SaveFormat=Array
  Demux1 : Demux  Orientation=left  Outputs=3
  Inner Loop Controller : Subsystem
  Mux1 : Mux  Orientation=left  Inputs=2
  Non-Linear Dynamics : Subsystem
  Saturation : Subsystem
  attitude : Scope
      settings: YMin=-4  YMax=10  SaveName=ScopeData4
  pqr : Scope
      settings: YMin=-4  YMax=10  SaveName=ScopeData3
  velocity : Scope
      settings: YMin=-4  YMax=10  SaveName=ScopeData2
  x : Terminator
  xyz : Scope
      settings: YMin=-0.1  YMax=1.2
  y : Terminator
  Body vel : Outport
  Position : Outport  Port=2
  Velocity : Outport  Port=3
  Angular Rates : Outport  Port=4
  Euler Angles : Outport  Port=5
  Inner Loop State : Outport  Port=6
  wires:
  Inner Loop Controller/2(Inner Loop State) -> Inner Loop State/1
  Saturation/1(Sensed) -> Position/1
  Outer Loop Request/1 -> Attitude Request/1, Inner Loop Controller/1(Outer Loop Request)
  Demux1/1 -> y/1
  Demux1/2 -> x/1
  Demux1/3 -> Inner Loop Controller/3(z State)
  Mux1/1 -> Inner Loop Controller/2(Attitude State)
  Non-Linear Dynamics/3(Velocity) -> velocity/1, Velocity/1  "xdot,ydot,zdot"
  Non-Linear Dynamics/4(Angular Rates) -> pqr/1, Mux1/2, Angular Rates/1  "p,q,r"
  Non-Linear Dynamics/5(Euler Angles) -> attitude/1, Mux1/1, Euler Angles/1
  Inner Loop Controller/1(Thrust Command) -> Non-Linear Dynamics/1(Thrust Command 1-4)
  Non-Linear Dynamics/1("Body vel ") -> Body vel/1
  Non-Linear Dynamics/2(Position) -> Saturation/1(Actual), xyz/1, Demux1/1  "x,y,z"

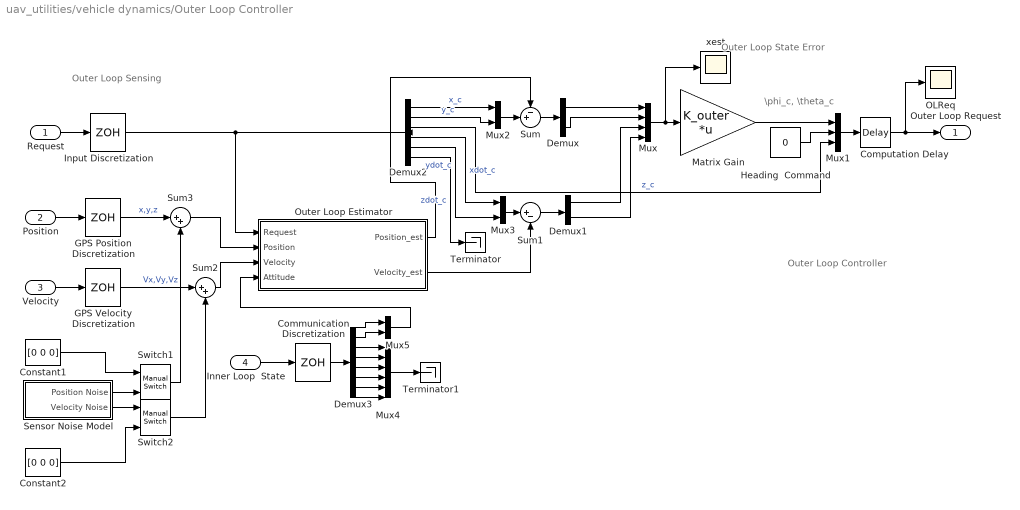
== system uav_utilities/vehicle dynamics/Outer Loop Controller ==
  note: Outer Loop Sensing
  note: Outer Loop
      | State Error
  note: \phi_c, \theta_c
  note: Outer Loop Controller
  Request : Inport
  Position : Inport  Port=2
  Velocity : Inport  Port=3
  Inner Loop  State : Inport  Port=4
  Communication Discretization : ZeroOrderHold  SampleTime=t_outer
  Computation Delay : TransportDelay  DelayTime=t_comp_outer
  Constant1 : Constant  Value=[0 0 0]
  Constant2 : Constant  Value=[0 0 0]
  Demux : Demux  Outputs=2
  Demux1 : Demux  Outputs=2
  Demux2 : Demux  Outputs=6
  Demux3 : Demux  Outputs=8
  GPS Position Discretization : ZeroOrderHold  SampleTime=t_gps
  GPS Velocity Discretization : ZeroOrderHold  SampleTime=t_gps
  Heading  Command : Constant  Value=0
  Input Discretization : ZeroOrderHold  SampleTime=t_outer
  Matrix Gain : Gain  Gain=K_outer  Multiplication=Matrix(K*u)  SaturateOnIntegerOverflow=on  OutDataTypeStr=Inherit: Same as input  ParamDataTypeStr=Inherit: Same as input
  Mux : Mux
  Mux1 : Mux  Inputs=3
  Mux2 : Mux  Inputs=2
  Mux3 : Mux  Inputs=2
  Mux4 : Mux  Inputs=6
  Mux5 : Mux  Inputs=2
  OLReq : Scope
      settings: YMin=-0.1  YMax=2  SaveName=ScopeData6
  Outer Loop Estimator : Subsystem
  "Sensor Noise Model " : Subsystem
  Sum : Sum  Inputs=-+|  SaturateOnIntegerOverflow=on
  Sum1 : Sum  Inputs=|+-  SaturateOnIntegerOverflow=on
  Sum2 : Sum  Inputs=|++  SaturateOnIntegerOverflow=on
  Sum3 : Sum  Inputs=|++  SaturateOnIntegerOverflow=on
  Switch1 : simulink/Signal Routing/Manual Switch  SystemSampleTime=-1  sw=1  action=0  varsize=off
  Switch2 : simulink/Signal Routing/Manual Switch  SystemSampleTime=-1  sw=0  action=0  varsize=off
  Terminator : Terminator
  Terminator1 : Terminator
  xest : Scope
      settings: YMin=-0.2  YMax=0.125  SaveName=ScopeData11
  Outer Loop Request : Outport
  wires:
  Communication Discretization/1 -> Demux3/1
  Constant1/1 -> Switch1/1
  Constant2/1 -> Switch2/2
  Switch1/1 -> Sum3/2
  "Sensor Noise Model "/1(Position Noise) -> Switch1/2
  Switch2/1 -> Sum2/2
  "Sensor Noise Model "/2(Velocity Noise) -> Switch2/1
  Sum3/1 -> Outer Loop Estimator/2(Position)
  Sum2/1 -> Outer Loop Estimator/3(Velocity)
  Mux5/1 -> Outer Loop Estimator/4(Attitude)
  Demux3/2 -> Mux5/2
  Demux3/1 -> Mux5/1
  Mux4/1 -> Terminator1/1
  Demux3/3 -> Mux4/1
  Demux3/4 -> Mux4/2
  Demux3/5 -> Mux4/3
  Demux3/6 -> Mux4/4
  Demux3/7 -> Mux4/5
  Demux3/8 -> Mux4/6
  Inner Loop  State/1 -> Communication Discretization/1
  Mux/1 -> xest/1, Matrix Gain/1
  Heading  Command/1 -> Mux1/2
  Computation Delay/1 -> OLReq/1, Outer Loop Request/1
  Mux1/1 -> Computation Delay/1
  Matrix Gain/1 -> Mux1/1
  Outer Loop Estimator/1(Position_est) -> Sum/1
  Mux2/1 -> Sum/2
  Outer Loop Estimator/2(Velocity_est) -> Sum1/2
  GPS Velocity Discretization/1 -> Sum2/1  "Vx,Vy,Vz"
  GPS Position Discretization/1 -> Sum3/1  "x,y,z"
  Demux2/6 -> Terminator/1  "zdot_c"
  Demux2/2 -> Mux2/2  "y_c"
  Demux2/1 -> Mux2/1  "x_c"
  Input Discretization/1 -> Outer Loop Estimator/1(Request), Demux2/1
  Demux2/5 -> Mux3/2  "ydot_c"
  Demux2/4 -> Mux3/1  "xdot_c"
  Demux2/3 -> Mux1/3  "z_c"
  Mux3/1 -> Sum1/1
  Request/1 -> Input Discretization/1
  Demux1/2 -> Mux/4
  Demux1/1 -> Mux/3
  Demux/2 -> Mux/2
  Demux/1 -> Mux/1
  Sum/1 -> Demux/1
  Sum1/1 -> Demux1/1
  Velocity/1 -> GPS Velocity Discretization/1
  Position/1 -> GPS Position Discretization/1

== system uav_utilities/STARMAC/gum_stix/body_to_inertial ==
  euler : Inport
  Ab : Inport  Port=2
  Ab_to_Ae : Stateflow chart
  inertial_vel_and pos_est : Subsystem  mask{Ts=.01}
      mask prompts: Ts "Sample Time [Ts] (seconds):"
  Xe : Outport
  Ve : Outport  Port=2
  wires:
  inertial_vel_and pos_est/2(Xb) -> Xe/1
  inertial_vel_and pos_est/1(Vb) -> Ve/1
  Ab_to_Ae/1(Ae) -> inertial_vel_and pos_est/1(Ab)
  Ab/1 -> Ab_to_Ae/2(Ab)
  euler/1 -> Ab_to_Ae/1(euler)

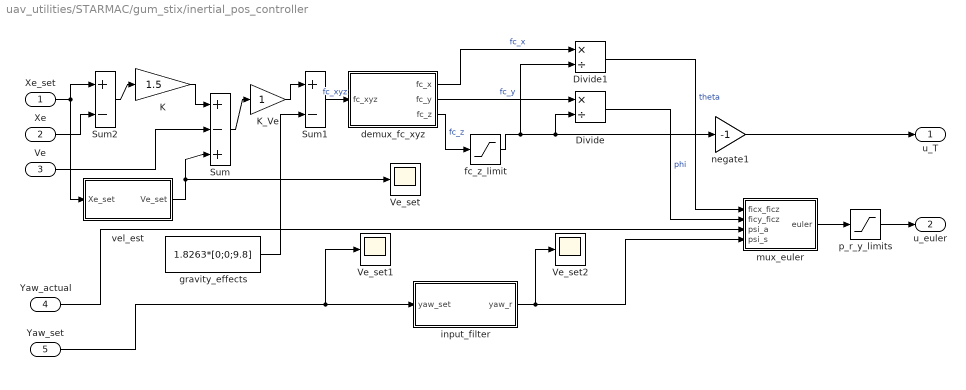
== system uav_utilities/STARMAC/gum_stix/inertial_pos_controller ==
  Xe_set : Inport
  Xe : Inport  Port=2
  Ve : Inport  Port=3
  Yaw_actual : Inport  Port=4
  Yaw_set : Inport  Port=5
  Divide : Product  Inputs=*/  OutDataTypeMode=single  OutDataType=sfix(16)  OutScaling=2^-10  OutDataTypeStr=single
  Divide1 : Product  Inputs=*/  OutDataTypeMode=single  OutDataType=sfix(16)  OutScaling=2^-10  OutDataTypeStr=single
  K : Gain  Gain=1.5  ParameterDataType=sfix(16)  ParameterScaling=2^0  OutDataTypeMode=single  OutDataType=sfix(16)  OutScaling=2^0  OutDataTypeStr=single
  K_Ve : Gain  ParameterDataTypeMode=single  ParameterDataType=sfix(16)  ParameterScaling=2^0  ParamDataTypeStr=single  OutDataTypeMode=single  OutDataType=sfix(16)  OutScaling=2^0  OutDataTypeStr=single
  Sum : Sum  Inputs=|+-+  AccumDataTypeStr=single  OutDataTypeMode=single  OutDataType=sfix(16)  OutScaling=2^0  OutDataTypeStr=single
  Sum1 : Sum  Inputs=|+-  AccumDataTypeStr=single  OutDataTypeMode=single  OutDataType=sfix(16)  OutScaling=2^0  OutDataTypeStr=single
  Sum2 : Sum  Inputs=|+-  AccumDataTypeStr=single  OutDataTypeMode=single  OutDataType=sfix(16)  OutScaling=2^0  OutDataTypeStr=single
  Ve_set : Scope
      settings: TimeRange=60  YMin=-1.75  YMax=2.25  SaveName=ScopeData2  Decimation=10
  Ve_set1 : Scope
      settings: TimeRange=60  SaveName=ScopeData10  Decimation=10
  Ve_set2 : Scope
      settings: TimeRange=60  SaveName=ScopeData11  Decimation=10
  demux_fc_xyz : Stateflow chart
  fc_z_limit : Saturate  UpperLimit=-(1/8)*9.81  LowerLimit=-4*9.81  OutDataTypeMode=single  OutDataType=sfix(16)  OutScaling=2^0  OutDataTypeStr=single
  gravity_effects : Constant  Value=1.8263*[0;0;9.8]  OutDataTypeMode=single  OutDataType=sfix(16)  OutScaling=2^0  OutDataTypeStr=single
  input_filter : Subsystem  mask{wn=1, zeta=0.9, T=0.01}
      mask prompts: wn "omega_n"; T "Sample time"
      mask init:
      | Hs=tf([wn^2],[1,2*zeta*wn,wn^2]);
      | Hz=ipesh_transform(Hs,T);
  mux_euler : Stateflow chart
  negate1 : Gain  Gain=-1  ParameterDataType=sfix(16)  ParameterScaling=2^0  OutDataTypeMode=single  OutDataType=sfix(16)  OutScaling=2^0  OutDataTypeStr=single
  p_r_y_limits : Saturate  UpperLimit=[pi/4,pi/4,inf]  LowerLimit=-[pi/4,pi/4,inf]  OutDataTypeMode=single  OutDataType=sfix(16)  OutScaling=2^0  OutDataTypeStr=single
  vel_est : Subsystem  mask{tau_f=.01/pi, T=.01}
      mask prompts: T "sample rate"
      mask init:
      | %b=1/tau_f;
      | %num1=(1-exp(-b*T));
      | %num2=-num1;
      | %den1=1;
      | %den2=-exp(-b*T);
      | %num=(1/T)*[num1 num2];
      | %den=[den1 den2];
      | %vel_est_a_1=single(-den(2)/den(1))
      | %vel_est_b_1=single(num(2)/den(1))
      | %vel_est_b_2=single(num(1)/den(1))
      | Hs=tf([1 0],[T/pi 1]);
      | Hz=ipesh_transform(Hs,T);
      | %Hz=tf(num,den,T);
      | %bode(Hz);
      | %hold on;
      | %bode(tf([1 0],[tau_f 1]));
  u_T : Outport
  u_euler : Outport  Port=2
  wires:
  Yaw_actual/1 -> mux_euler/3(psi_a)
  Yaw_set/1 -> Ve_set1/1, input_filter/1(yaw_set)
  input_filter/1(yaw_r) -> mux_euler/4(psi_s), Ve_set2/1
  Divide/1 -> mux_euler/2(ficy_ficz)  "phi"
  Divide1/1 -> mux_euler/1(ficx_ficz)  "theta"
  vel_est/1(Ve_set) -> Ve_set/1, Sum/3
  Ve/1 -> Sum/2
  K_Ve/1 -> Sum1/1
  demux_fc_xyz/2(fc_y) -> Divide/1  "fc_y"
  K/1 -> Sum/1
  Sum2/1 -> K/1
  Xe/1 -> Sum2/2
  Sum/1 -> K_Ve/1
  gravity_effects/1 -> Sum1/2
  Sum1/1 -> demux_fc_xyz/1(fc_xyz)  "fc_xyz"
  mux_euler/1(euler) -> p_r_y_limits/1
  demux_fc_xyz/3(fc_z) -> fc_z_limit/1  "fc_z"
  demux_fc_xyz/1(fc_x) -> Divide1/1  "fc_x"
  p_r_y_limits/1 -> u_euler/1
  negate1/1 -> u_T/1
  Xe_set/1 -> vel_est/1(Xe_set), Sum2/1
  fc_z_limit/1 -> negate1/1, Divide/2, Divide1/2

== system uav_utilities/STARMAC/gum_stix/rate_limiter ==
  Xe_set : Inport  OutDataType=sfix(16)  OutScaling=2^0
  Constant : Constant  Value=T  OutDataTypeMode=single  OutDataType=sfix(16)  OutScaling=2^0  OutDataTypeStr=single
  Constant1 : Constant  Value=Vmax  OutDataTypeMode=single  OutDataType=sfix(16)  OutScaling=2^0  OutDataTypeStr=single
  Demux : Demux  Outputs=3
  Discrete Transfer Fcn : DiscreteTransferFcn  Numerator=Hz.num{1}  Denominator=Hz.den{1}  SampleTime=-1
  Discrete Transfer Fcn1 : DiscreteTransferFcn  Numerator=Hz.num{1}  Denominator=Hz.den{1}  SampleTime=-1
  Discrete Transfer Fcn2 : DiscreteTransferFcn  Numerator=Hz.num{1}  Denominator=Hz.den{1}  SampleTime=-1
  Embedded MATLAB Function : Stateflow chart
  Mux : Mux  Inputs=3
  Unit Delay : UnitDelay  Orientation=left  SampleTime=-1
  Xr_set : Outport  OutDataType=sfix(16)  OutScaling=2^0
  wires:
  Discrete Transfer Fcn2/1 -> Mux/3
  Demux/3 -> Discrete Transfer Fcn2/1
  Discrete Transfer Fcn1/1 -> Mux/2
  Demux/2 -> Discrete Transfer Fcn1/1
  Discrete Transfer Fcn/1 -> Mux/1
  Demux/1 -> Discrete Transfer Fcn/1
  Constant1/1 -> Embedded MATLAB Function/4(Vmax)
  Constant/1 -> Embedded MATLAB Function/3(Tsamp)
  Unit Delay/1 -> Embedded MATLAB Function/2(Xd_prev)
  Embedded MATLAB Function/1(Xr) -> Unit Delay/1, Xr_set/1
  Mux/1 -> Embedded MATLAB Function/1(Xd)
  Xe_set/1 -> Demux/1

== system uav_utilities/STARMAC/gum_stix/sensor_fusion ==
  Xe_f : Inport
  Ve_f : Inport  Port=2
  Xe_s : Inport  Port=3
  Ve_s : Inport  Port=4
  Sum : Sum  Inputs=|+-  OutDataTypeMode=single  OutDataType=sfix(16)  OutScaling=2^0  OutDataTypeStr=single
  Sum1 : Sum  Inputs=|+-  OutDataTypeMode=single  OutDataType=sfix(16)  OutScaling=2^0  OutDataTypeStr=single
  delays : Subsystem  Orientation=left
  if_end : Subsystem
  if_end1 : Subsystem
  Xe : Outport
  Ve : Outport  Port=2
  wires:
  Sum1/1 -> Ve/1
  Sum/1 -> Xe/1
  if_end/1(Xe_sh_1) -> delays/4(Xe_sh)
  if_end1/1(Ve_sh_1) -> delays/3(Ve_sh)
  if_end1/2(dV_1) -> Sum1/2, delays/1(dV)
  if_end/2(dX_1) -> Sum/2, delays/2(dX)
  delays/3(Ve_sh_1) -> if_end1/4(Ve_sh_1p)
  delays/1(dV_1) -> if_end1/3(dV_1p)
  Ve_s/1 -> if_end1/1(Ve_s)
  Ve_f/1 -> Sum1/1, if_end1/2(Ve_f)
  delays/4(Xe_sh_1) -> if_end/4(Xe_sh_1p)
  Xe_s/1 -> if_end/1(Xe_s)
  delays/2(dX_1) -> if_end/3(dX_1p)
  Xe_f/1 -> Sum/1, if_end/2(Xe_f)

== system uav_utilities/STARMAC/robo_stix/euler_controller ==
  euler_set : Inport
  euler : Inport  Port=2
  omega : Inport  Port=3
  K_euler : Gain  Gain=single(K_e)  ParameterDataType=sfix(16)  ParameterScaling=2^0  OutDataType=sfix(16)  OutScaling=2^0
  K_omega : Gain  Gain=single(K_o)  ParameterDataType=sfix(16)  ParameterScaling=2^0  OutDataTypeMode=single  OutDataType=sfix(16)  OutScaling=2^0  OutDataTypeStr=single
  Sum : Sum  Inputs=|+-  AccumDataTypeStr=single  OutDataType=sfix(16)  OutScaling=2^0
  Sum1 : Sum  Inputs=|+-  AccumDataTypeStr=single  OutDataType=sfix(16)  OutScaling=2^0
  euler_set_euler_omega_u_omega : Scope  NumInputPorts=4
      settings: YMin=-7~-7~-0.3~-0.3  YMax=1~1~0.3~0.3  SaveName=ScopeData8  Decimation=10
  torque_limit : Saturate  UpperLimit=9.8*.3048*ones(3,1)  LowerLimit=-9.8*.3048*ones(3,1)  OutDataTypeMode=single  OutDataType=sfix(16)  OutScaling=2^0  OutDataTypeStr=single
  u_torque : Outport
  wires:
  omega/1 -> euler_set_euler_omega_u_omega/3, Sum/2  "omega"
  K_omega/1 -> torque_limit/1
  torque_limit/1 -> u_torque/1
  K_euler/1 -> euler_set_euler_omega_u_omega/4, Sum/1  "u_omega"
  euler/1 -> euler_set_euler_omega_u_omega/2, Sum1/2  "euler"
  Sum1/1 -> K_euler/1
  euler_set/1 -> euler_set_euler_omega_u_omega/1, Sum1/1  "euler_set"
  Sum/1 -> K_omega/1

== system uav_utilities/STARMAC/robo_stix/lead_motor ==
  thrust_in : Inport  DataType=single  OutDataTypeStr=single
  Demux : Demux
  Discrete Transfer Fcn{,1..3} (4 alike) : DiscreteTransferFcn  Numerator=Hz.num{1}  Denominator=Hz.den{1}  SampleTime=-1
  Mux : Mux
  thrust_out : Outport  DataType=single  OutDataTypeStr=single
  wires:
  Discrete Transfer Fcn3/1 -> Mux/4
  Demux/4 -> Discrete Transfer Fcn3/1
  Discrete Transfer Fcn2/1 -> Mux/3
  Discrete Transfer Fcn1/1 -> Mux/2
  Discrete Transfer Fcn/1 -> Mux/1
  Mux/1 -> thrust_out/1
  Demux/3 -> Discrete Transfer Fcn2/1
  Demux/2 -> Discrete Transfer Fcn1/1
  Demux/1 -> Discrete Transfer Fcn/1
  thrust_in/1 -> Demux/1  "x"

== system uav_utilities/STARMAC/robo_stix/sensor_convert ==
  euler_s : Inport
  Ab_s : Inport  Port=2
  omega_s : Inport  Port=3
  accel_per_count : Gain  Gain=(9.81*a_g_s)/(1e3*32768)  ParameterDataType=sfix(16)  ParameterScaling=2^0  OutDataTypeMode=single  OutDataType=sfix(16)  OutScaling=2^0  OutDataTypeStr=single
  radian_p_sec_per_count : Gain  Gain=g_g_s/(1e3*32768)  ParameterDataType=sfix(16)  ParameterScaling=2^0  OutDataTypeMode=single  OutDataType=sfix(16)  OutScaling=2^0  OutDataTypeStr=single
  radian_per_count : Gain  Gain=pi/32768  ParameterDataType=sfix(16)  ParameterScaling=2^0  OutDataTypeMode=single  OutDataType=sfix(16)  OutScaling=2^0  OutDataTypeStr=single
  euler : Outport
  Ab : Outport  Port=2
  omega : Outport  Port=3
  wires:
  radian_p_sec_per_count/1 -> omega/1
  omega_s/1 -> radian_p_sec_per_count/1
  accel_per_count/1 -> Ab/1
  Ab_s/1 -> accel_per_count/1
  radian_per_count/1 -> euler/1
  euler_s/1 -> radian_per_count/1

== system uav_utilities/STARMAC/robo_stix/u_T_u_torque_motor_thrust ==
  u_torque : Inport
  u_T : Inport  Port=2
  Mi : Gain  Gain=Mi  Multiplication=Matrix(K*u)  ParameterDataTypeMode=single  ParameterDataType=sfix(16)  ParameterScaling=2^0  ParamDataTypeStr=single  OutDataTypeMode=single  OutDataType=sfix(16)  OutScaling=2^0  OutDataTypeStr=single
  u_torque_u_T_mux : Stateflow chart
  cont_motor_thrust : Outport
  wires:
  u_torque_u_T_mux/1(u_torque_u_T) -> Mi/1
  Mi/1 -> cont_motor_thrust/1
  u_T/1 -> u_torque_u_T_mux/2(u_T)
  u_torque/1 -> u_torque_u_T_mux/1(u_torque)

== system uav_utilities/STARMAC/starmac_dynamics/6DOF_Euler_Angles ==
  note: 6 DOF System Model
  note: This subsystem models a 6 degree of freedom (6DOF) system in Euler angles.
      | A Direct Cosine Matrix (DCM) is produced to allow for easy transformations to
      | and from the reference frame of the body.  Enter appropriate Parameters in the dialog menu.
      | Follows Euler Angle Sequence (1,2,3), see Section 5.6, Representing Attitude: Euler Angles, Unit
      | Quaternions, and Rotation by James Diebel.  Interface matches that from the Aerospace Toolbox
      | for non variable mass (6DoF EoM (Body Axis) for Euler Angles).
      |
      | J. Kapinski
      | Carnegia Mellon University
      | 7/2007
      | Revised:
      | Nicholas Kottenstette, ISIS, 8/2008
  F_xyz(N) : Inport  OutDataType=sfix(16)  OutScaling=2^0
  M_xyz(Nm) : Inport  Port=2  PortDimensions=3  OutDataType=sfix(16)  OutScaling=2^0
  body_euler_to_earth : aero_sim_lib/body_euler_to_earth  SystemSampleTime=-1  XYZe_0=XYZe_0
  continuous_body_dynamics : aero_sim_lib/continuous_body_dynamics  SystemSampleTime=-1  M=M  Vb_0=Vb_0
  continuous_inertia_body_dynamics : aero_sim_lib/continuous_inertia_body_dynamics  SystemSampleTime=-1  I=I  omega_0=omega_0
  omega_to_euler : aero_sim_lib/omega_to_euler  SystemSampleTime=-1  euler_0=euler_0
  Ve : Outport  OutDataType=sfix(16)  OutScaling=2^0
  Xe : Outport  Port=2  OutDataType=sfix(16)  OutScaling=2^0
  euler : Outport  Port=3  OutDataType=sfix(16)  OutScaling=2^0
  DCM : Outport  Port=4  OutDataType=sfix(16)  OutScaling=2^0
  Vb : Outport  Port=5  OutDataType=sfix(16)  OutScaling=2^0
  omega : Outport  Port=6  OutDataType=sfix(16)  OutScaling=2^0
  domega/dt : Outport  Port=7  OutDataType=sfix(16)  OutScaling=2^0
  Ab : Outport  Port=8  OutDataType=sfix(16)  OutScaling=2^0
  wires:
  M_xyz(Nm)/1 -> continuous_inertia_body_dynamics/1
  F_xyz(N)/1 -> continuous_body_dynamics/1
  continuous_inertia_body_dynamics/1 -> omega/1, continuous_body_dynamics/2, omega_to_euler/1
  continuous_body_dynamics/1 -> Vb/1, body_euler_to_earth/2
  continuous_body_dynamics/2 -> Ab/1
  continuous_inertia_body_dynamics/2 -> domega/dt/1
  omega_to_euler/1 -> euler/1, body_euler_to_earth/1
  body_euler_to_earth/1 -> Ve/1
  body_euler_to_earth/2 -> DCM/1
  body_euler_to_earth/3 -> Xe/1

== system uav_utilities/STARMAC/starmac_dynamics/starmac_blade_flapping_effects ==
  motor_thrusts : Inport  OutDataType=sfix(16)  OutScaling=2^0
  v_body_relative : Inport  Port=2  OutDataType=sfix(16)  OutScaling=2^0
  Pick First 2 Elements : Constant  Value=[1 0 0; 0 1 0; 0 0 0]  OutDataType=sfix(16)  OutScaling=2^0
  Product : Product  OutDataType=sfix(16)  OutScaling=2^0  RndMeth=Zero
  Product2 : Product  Multiplication=Matrix(*)  OutDataType=sfix(16)  OutScaling=2^0  RndMeth=Zero
  Product4 : Product  OutDataType=sfix(16)  OutScaling=2^0  RndMeth=Zero
  Sum : Sum  Inputs=|++  OutDataType=sfix(16)  OutScaling=2^0
  Sum of Elements : Sum  Inputs=+  OutDataType=sfix(16)  OutScaling=2^-10
  starmac_body_moments : Subsystem  AncestorBlock=aero_sim_lib/starmac_body_moments  mask{dx=.3048, dz=.07, K_torque=.47}
  starmac_flapping_dynamics : Subsystem  AncestorBlock=aero_sim_lib/starmac_flapping_dynamics  mask{K_a1s=.009, K_beta=.23}
  starmac_vertical_effect_dynamics : Subsystem  AncestorBlock=aero_sim_lib/starmac_vertical_effect_dynamics  mask{tau_motor=0.1, R=0.127, Alpha=(pi/180)*[-85:5:85], Vinf=[0:0.5:6], Thrust=9.8*[0.3:0.02:0.8]}
      mask prompts: tau_motor "motor time constant (s)"; R "radius of propeller (m)"; Alpha "Alpha (radians)"; Vinf "Vinf (radians)"; Thrust "Propeller Thrust (N)"
      mask init:
      | rho = 1.2;
      | A = pi*R^2;
      | Vh = sqrt(Thrust/(2*rho*A));
      | for i = 1:length(Vh)
      |     for j = 1:length(Vinf)
      |         for k = 1:length(Alpha)
      |             Vi(k,j,i) = find_vi(Vh(i),Vinf(j),Alpha(k));
      |             ToverTh(k,j,i) = min(10,max(0.1,Vh(i)/(Vi(k,j,i)+Vinf(j)*sin(Alpha(k)))));
      |         end
      |     end
      | end
  body_forces : Outport  OutDataType=sfix(16)  OutScaling=2^0
  body_moments : Outport  Port=2  OutDataType=sfix(16)  OutScaling=2^0
  wires:
  Product/1 -> starmac_body_moments/1(Thrust Magnitudes), Sum of Elements/1
  starmac_vertical_effect_dynamics/1(thrust_multiplier) -> Product/2
  motor_thrusts/1 -> starmac_vertical_effect_dynamics/1(motor_thrusts), Product/1
  Pick First 2 Elements/1 -> Product2/1
  v_body_relative/1 -> starmac_vertical_effect_dynamics/2(v_body_relative), Product2/2
  Product2/1 -> starmac_flapping_dynamics/1(Vb2_hat)
  Sum of Elements/1 -> Product4/1
  Product4/1 -> body_forces/1
  starmac_flapping_dynamics/1(thrust_vector) -> starmac_body_moments/2(Thrust Vector), Product4/2
  starmac_body_moments/1(Body Moments) -> Sum/1
  Sum/1 -> body_moments/1
  starmac_flapping_dynamics/2(rotor_blade_moments) -> Sum/2
